simulink model "AD_Vehicle_part10"  (R2021a)
settings: Solver=VariableStepAuto  StartTime=0.0  StopTime=20  RelTol=1e-3
libraries: vrlib x2, mpcadaslib x1, pid_lib x1, simulink x1
settings Model: SimulationMode=accelerator  Creator=admin  LastModifiedBy=admin

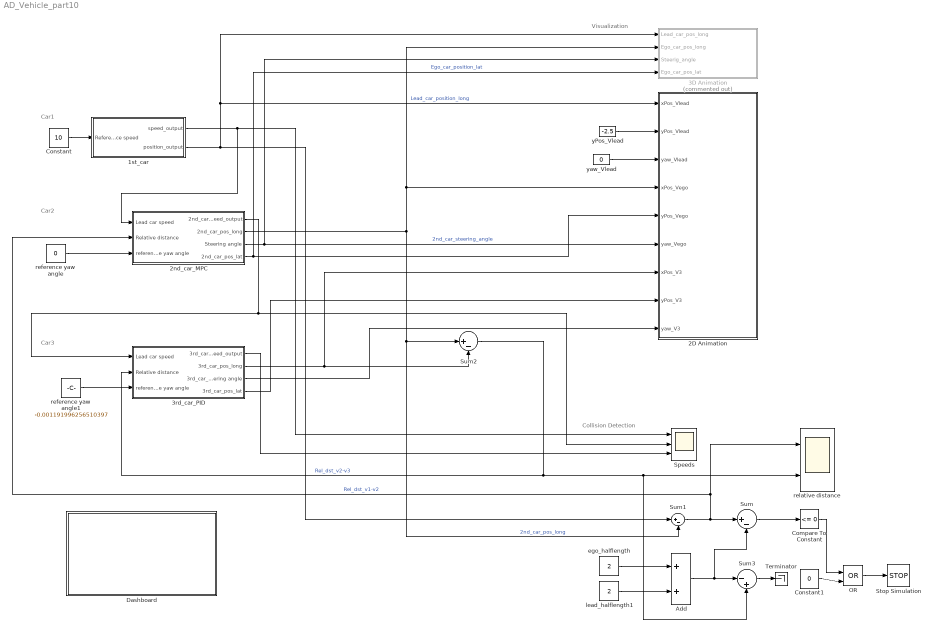
== system AD_Vehicle_part10 ==
  note: Car3
  note: Car2
  note: Car1
  note: Visualization
  note: Collision Detection
  1st_car : Subsystem  mask{Pos=40, Speed=20}
      mask prompts: Pos "Initial Position"; Speed "Initial Speed"
      mask TypeOptions Pos: initial_position/Value
      mask TypeOptions Speed: initial_speed/Value
  2D Animation : Subsystem  TreatAsAtomicUnit=on  SystemSampleTime=0.02
  2nd_car_MPC : Subsystem  mask{Pos_Z=20, Speed=25, Pos_X=-2.5}
      mask prompts: Pos_Z "Initial Position longi"; Speed "Initial Speed"; Pos_X "Initial position lat"
      mask TypeOptions Pos_Z: initial_position_long/Value
      mask TypeOptions Speed: initial_speed/Value
      mask TypeOptions Pos_X: initial_position_lat/Value
  3D Animation : Subsystem  Commented=on
  3rd_car_PID : Subsystem  mask{Pos_Z=0, Speed=20, Pos_X=-2.5}
      mask prompts: Pos_Z "Initial Position longi"; Speed "Initial Speed"; Pos_X "Initial position lat"
      mask TypeOptions Pos_Z: initial_position_long/Value
      mask TypeOptions Speed: initial_speed/Value
      mask TypeOptions Pos_X: initial_position_lat/Value
  Add : Sum
  Compare To Constant : simulink/Logic and Bit Operations/Compare To Constant  relop=<=  const=0  OutDataTypeStr=boolean
  Constant : Constant  Value=10
  Constant1 : Constant  Value=0
  Dashboard : Subsystem
  OR : Logic  Operator=OR  IconShape=distinctive  AllPortsSameDT=off  OutDataTypeStr=boolean
  Speeds : Scope  NumInputPorts=3
  Stop Simulation : Stop
  Sum : Sum  Inputs=|+-
  Sum1 : Sum  Inputs=|+-
  Sum2 : Sum  Inputs=|+-
  Sum3 : Sum  Inputs=|-+
  Terminator : Terminator
  ego_halflength : Constant  Value=2
  lead_halflength1 : Constant  Value=2
  reference yaw angle : Constant  Value=0
  reference yaw angle1 : Constant  Value=-0.001191996256510397
  relative distance : Scope  NumInputPorts=2
  yPos_Vlead : Constant  Value=-2.5
  yaw_Vlead : Constant  Value=0
  wires:
  3rd_car_PID/2(3rd_car_pos_long) -> 2D Animation/7(xPos_V3), Sum2/2
  Sum/1 -> Compare To Constant/1
  Constant/1 -> 1st_car/1(Reference speed)
  Sum2/1 -> Sum3/2, relative distance/2, 3rd_car_PID/2(Relative distance)  "Rel_dst_v2-v3"
  2nd_car_MPC/1(2nd_car_speed_output) -> 3rd_car_PID/1(Lead car speed), Speeds/2
  reference yaw angle1/1 -> 3rd_car_PID/3(reference yaw angle)
  2nd_car_MPC/4(2nd_car_pos_lat) -> 3D Animation/4(Ego_car_pos_lat), 2D Animation/5(yPos_Vego)  "Ego_car_position_lat"
  reference yaw angle/1 -> 2nd_car_MPC/3(reference yaw angle)
  Sum1/1 -> 2nd_car_MPC/2(Relative distance), relative distance/1, Sum/1  "Rel_dst_v1-v2"
  2nd_car_MPC/3(Steering angle) -> 3D Animation/3(Steerig_angle), 2D Animation/6(yaw_Vego)  "2nd_car_steering_angle"
  lead_halflength1/1 -> Add/2
  2nd_car_MPC/2(2nd_car_pos_long) -> Sum1/2, Sum2/1, 2D Animation/4(xPos_Vego), 3D Animation/2(Ego_car_pos_long)  "2nd_car_pos_long"
  yaw_Vlead/1 -> 2D Animation/3(yaw_Vlead)
  yPos_Vlead/1 -> 2D Animation/2(yPos_Vlead)
  1st_car/2(position_output) -> 3D Animation/1(Lead_car_pos_long), 2D Animation/1(xPos_Vlead), Sum1/1  "Lead_car_position_long"
  1st_car/1(speed_output) -> Speeds/1, 2nd_car_MPC/1(Lead car speed)
  Constant1/1 -> OR/2
  Sum3/1 -> Terminator/1
  Compare To Constant/1 -> OR/1
  Add/1 -> Sum3/1, Sum/2
  OR/1 -> Stop Simulation/1
  ego_halflength/1 -> Add/1
  3rd_car_PID/1(3rd_car_speed_output) -> Speeds/3
  3rd_car_PID/4(3rd_car_pos_lat) -> 2D Animation/8(yPos_V3)
  3rd_car_PID/3(3rd_car_Steering angle) -> 2D Animation/9(yaw_V3)

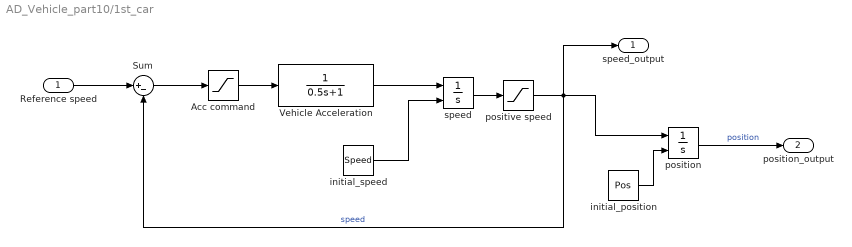
== system AD_Vehicle_part10/1st_car ==
  Reference speed : Inport
  Acc command : Saturate  UpperLimit=2  LowerLimit=-3
  Sum : Sum  Inputs=|+-
  Vehicle Acceleration : TransferFcn  Denominator=[0.5 1]
  initial_position : Constant  Value=Pos
  initial_speed : Constant  Value=Speed
  position : Integrator  InitialConditionSource=external
  positive speed : Saturate  UpperLimit=220  LowerLimit=0
  speed : Integrator  InitialConditionSource=external
  speed_output : Outport
  position_output : Outport  Port=2
  wires:
  Acc command/1 -> Vehicle Acceleration/1
  positive speed/1 -> speed_output/1, Sum/2, position/1  "speed"
  position/1 -> position_output/1  "position"
  speed/1 -> positive speed/1
  initial_position/1 -> position/2
  Sum/1 -> Acc command/1
  initial_speed/1 -> speed/2
  Reference speed/1 -> Sum/1
  Vehicle Acceleration/1 -> speed/1

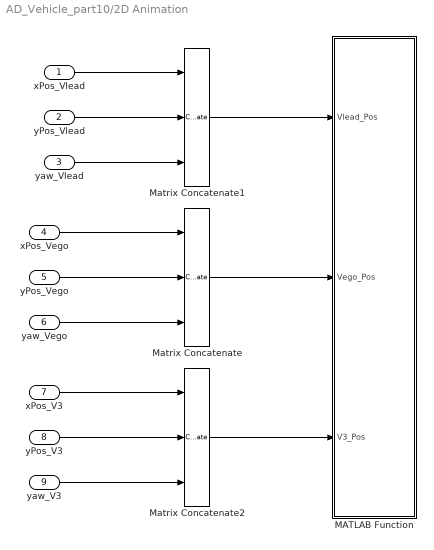
== system AD_Vehicle_part10/2D Animation ==
  xPos_Vlead : Inport
  yPos_Vlead : Inport  Port=2
  yaw_Vlead : Inport  Port=3
  xPos_Vego : Inport  Port=4
  yPos_Vego : Inport  Port=5
  yaw_Vego : Inport  Port=6
  xPos_V3 : Inport  Port=7
  yPos_V3 : Inport  Port=8
  yaw_V3 : Inport  Port=9
  MATLAB Function : MATLAB Function  TreatAsAtomicUnit=on
      mask init:
      | close all;
      | figure('units','normalized','outerposition',[0.5 0 0.5 1]); % 设置窗口(figure)位置大小
      | set (gca,'units','normalized','position',[0.1,0.3,0.9,0.5] ); % 设置画布(axis)大小位置
      | grid on;
      | axis equal;
      | hold on;
  Matrix Concatenate : Concatenate  NumInputs=3  ConcatenateDimension=2
  Matrix Concatenate1 : Concatenate  NumInputs=3  ConcatenateDimension=2
  Matrix Concatenate2 : Concatenate  NumInputs=3  ConcatenateDimension=2
  wires:
  Matrix Concatenate/1 -> MATLAB Function/2(Vego_Pos)
  yPos_Vego/1 -> Matrix Concatenate/2
  xPos_Vego/1 -> Matrix Concatenate/1
  yaw_Vego/1 -> Matrix Concatenate/3
  Matrix Concatenate1/1 -> MATLAB Function/1(Vlead_Pos)
  yPos_Vlead/1 -> Matrix Concatenate1/2
  xPos_Vlead/1 -> Matrix Concatenate1/1
  yaw_Vlead/1 -> Matrix Concatenate1/3
  xPos_V3/1 -> Matrix Concatenate2/1
  yPos_V3/1 -> Matrix Concatenate2/2
  yaw_V3/1 -> Matrix Concatenate2/3
  Matrix Concatenate2/1 -> MATLAB Function/3(V3_Pos)

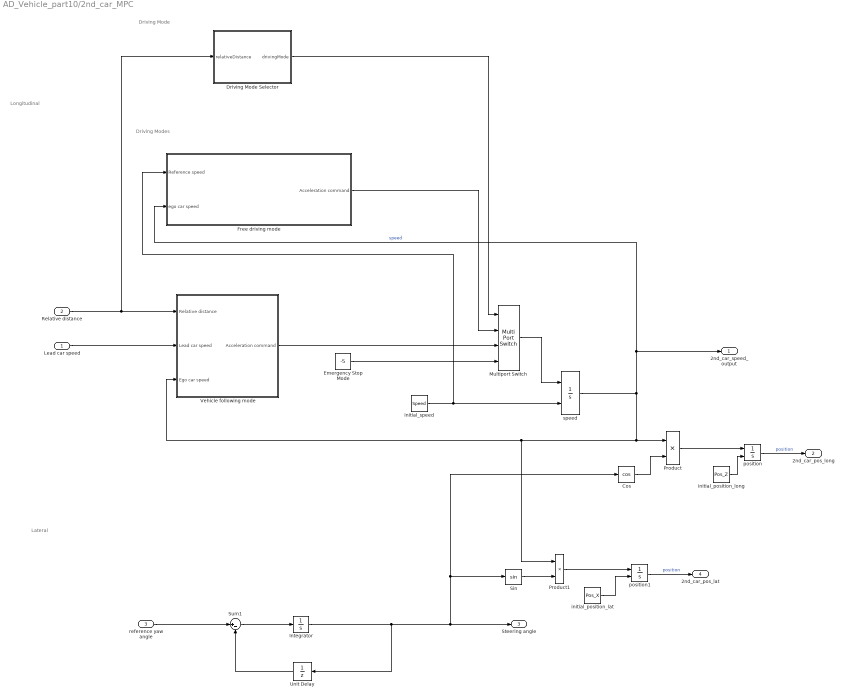
== system AD_Vehicle_part10/2nd_car_MPC ==
  note: Driving Mode
  note: Driving Modes
  note: Lateral
  note: Longitudinal
  Lead car speed : Inport
  Relative distance : Inport  Port=2
  reference yaw angle : Inport  Port=3
  Cos : Trigonometry  Operator=cos
  Driving Mode Selector : Stateflow chart  TreatAsAtomicUnit=on
  Emergency Stop Mode : Constant  Value=-5
  Free driving mode : Subsystem
  Integrator : Integrator
  Multiport Switch : MultiPortSwitch
  Product : Product
  Product1 : Product
  Sin : Trigonometry
  Sum1 : Sum  Inputs=|+-
  Unit Delay : UnitDelay  SampleTime=-1  HasFrameUpgradeWarning=on
  Vehicle following mode : Subsystem
  initial_position_lat : Constant  Value=Pos_X
  initial_position_long : Constant  Value=Pos_Z
  initial_speed : Constant  Value=Speed
  position : Integrator  InitialConditionSource=external
  position1 : Integrator  InitialConditionSource=external
  speed : Integrator  InitialConditionSource=external  LimitOutput=on  LowerSaturationLimit=0
  2nd_car_speed_output : Outport
  2nd_car_pos_long : Outport  Port=2
  Steering angle : Outport  Port=3
  2nd_car_pos_lat : Outport  Port=4
  wires:
  speed/1 -> Free driving mode/2("ego car speed "), 2nd_car_speed_output/1, Product1/1, Vehicle following mode/3(Ego car speed), Product/1  "speed"
  position/1 -> 2nd_car_pos_long/1  "position"
  initial_position_long/1 -> position/2
  initial_speed/1 -> speed/2, Free driving mode/1(Reference speed)
  Integrator/1 -> Unit Delay/1, Sin/1, Cos/1, Steering angle/1
  reference yaw angle/1 -> Sum1/1
  Sum1/1 -> Integrator/1
  Unit Delay/1 -> Sum1/2
  initial_position_lat/1 -> position1/2
  position1/1 -> 2nd_car_pos_lat/1  "position"
  Product/1 -> position/1
  Cos/1 -> Product/2
  Product1/1 -> position1/1
  Sin/1 -> Product1/2
  Relative distance/1 -> Vehicle following mode/1(Relative distance), Driving Mode Selector/1(relativeDistance)
  Lead car speed/1 -> Vehicle following mode/2(Lead car speed)
  Vehicle following mode/1(Acceleration command) -> Multiport Switch/3
  Multiport Switch/1 -> speed/1
  Free driving mode/1(Acceleration command) -> Multiport Switch/2
  Emergency Stop Mode/1 -> Multiport Switch/4
  Driving Mode Selector/1(drivingMode) -> Multiport Switch/1

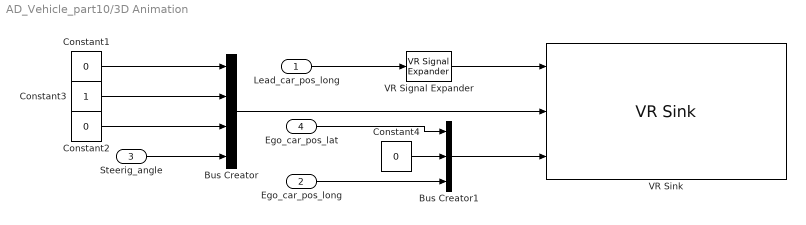
== system AD_Vehicle_part10/3D Animation ==
  Lead_car_pos_long : Inport
  Ego_car_pos_long : Inport  Port=2
  Steerig_angle : Inport  Port=3
  Ego_car_pos_lat : Inport  Port=4
  Bus Creator : BusCreator  Inputs=4
  Bus Creator1 : BusCreator  Inputs=3
  Constant1 : Constant  Value=0
  Constant2 : Constant  Value=0
  Constant3 : Constant
  Constant4 : Constant  Value=0
  VR Signal Expander : vrlib/VR Signal Expander  outwidth=3  outidx=[3]
  VR Sink : vrlib/VR Sink  InstantiateOnLoad=on  SampleTime=0.05  ViewEnable=on  RemoteChange=off  RemoteView=off  FieldsWritten=Car_Red.translation.3.1.1.double#Car_Blue.rotation.4.1.1.double#Car_Blue.translation.3.1.1.double  WorldFileName=PlatoonWorld.WRL  AutoView=off  VideoDimensions=[]  AllowVariableSize=off
  wires:
  Lead_car_pos_long/1 -> VR Signal Expander/1
  Constant4/1 -> Bus Creator1/2
  Bus Creator/1 -> VR Sink/2
  Constant1/1 -> Bus Creator/1
  Constant3/1 -> Bus Creator/2
  VR Signal Expander/1 -> VR Sink/1
  Ego_car_pos_long/1 -> Bus Creator1/3
  Bus Creator1/1 -> VR Sink/3
  Constant2/1 -> Bus Creator/3
  Ego_car_pos_lat/1 -> Bus Creator1/1
  Steerig_angle/1 -> Bus Creator/4

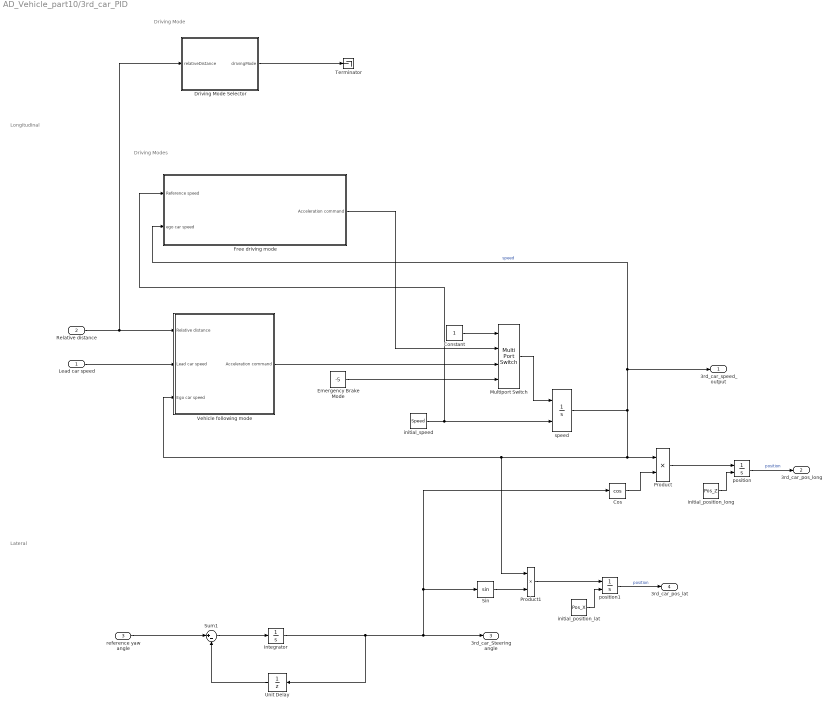
== system AD_Vehicle_part10/3rd_car_PID ==
  note: Driving Mode
  note: Driving Modes
  note: Lateral
  note: Longitudinal
  Lead car speed : Inport
  Relative distance : Inport  Port=2
  reference yaw angle : Inport  Port=3
  Constant : Constant
  Cos : Trigonometry  Operator=cos
  Driving Mode Selector : Stateflow chart  TreatAsAtomicUnit=on
  Emergency Brake Mode : Constant  Value=-5
  Free driving mode : Subsystem
  Integrator : Integrator
  Multiport Switch : MultiPortSwitch
  Product : Product
  Product1 : Product
  Sin : Trigonometry
  Sum1 : Sum  Inputs=|+-
  Terminator : Terminator
  Unit Delay : UnitDelay  SampleTime=-1  HasFrameUpgradeWarning=on
  Vehicle following mode : Subsystem
  initial_position_lat : Constant  Value=Pos_X
  initial_position_long : Constant  Value=Pos_Z
  initial_speed : Constant  Value=Speed
  position : Integrator  InitialConditionSource=external
  position1 : Integrator  InitialConditionSource=external
  speed : Integrator  InitialConditionSource=external  LimitOutput=on  LowerSaturationLimit=0
  3rd_car_speed_output : Outport
  3rd_car_pos_long : Outport  Port=2
  3rd_car_Steering angle : Outport  Port=3
  3rd_car_pos_lat : Outport  Port=4
  wires:
  speed/1 -> Free driving mode/2("ego car speed "), 3rd_car_speed_output/1, Product1/1, Vehicle following mode/3(Ego car speed), Product/1  "speed"
  position/1 -> 3rd_car_pos_long/1  "position"
  initial_position_long/1 -> position/2
  initial_speed/1 -> speed/2, Free driving mode/1(Reference speed)
  Integrator/1 -> Unit Delay/1, Sin/1, Cos/1, 3rd_car_Steering angle/1
  reference yaw angle/1 -> Sum1/1
  Sum1/1 -> Integrator/1
  Unit Delay/1 -> Sum1/2
  initial_position_lat/1 -> position1/2
  position1/1 -> 3rd_car_pos_lat/1  "position"
  Product/1 -> position/1
  Cos/1 -> Product/2
  Product1/1 -> position1/1
  Sin/1 -> Product1/2
  Relative distance/1 -> Vehicle following mode/1(Relative distance), Driving Mode Selector/1(relativeDistance)
  Lead car speed/1 -> Vehicle following mode/2(Lead car speed)
  Vehicle following mode/1(Acceleration command) -> Multiport Switch/3
  Multiport Switch/1 -> speed/1
  Free driving mode/1(Acceleration command) -> Multiport Switch/2
  Emergency Brake Mode/1 -> Multiport Switch/4
  Driving Mode Selector/1(drivingMode) -> Terminator/1
  Constant/1 -> Multiport Switch/1

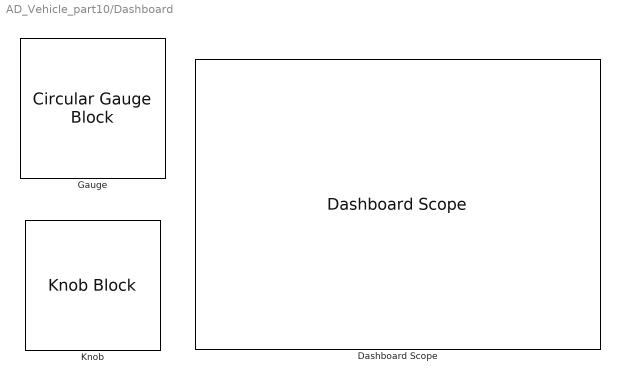
== system AD_Vehicle_part10/Dashboard ==
  Dashboard Scope : DashboardScope
  Gauge : CircularGaugeBlock  ScaleMax=180
  Knob : KnobBlock  ScaleMin=-0.2  ScaleMax=0.2

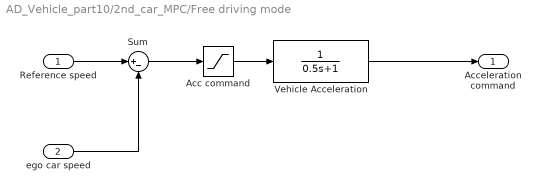
== system AD_Vehicle_part10/2nd_car_MPC/Free driving mode ==
  Reference speed : Inport
  "ego car speed " : Inport  Port=2
  Acc command : Saturate  UpperLimit=2  LowerLimit=-3
  Sum : Sum  Inputs=|+-
  Vehicle Acceleration : TransferFcn  Denominator=[0.5 1]
  Acceleration command : Outport
  wires:
  Vehicle Acceleration/1 -> Acceleration command/1
  Sum/1 -> Acc command/1
  Acc command/1 -> Vehicle Acceleration/1
  Reference speed/1 -> Sum/1
  "ego car speed "/1 -> Sum/2

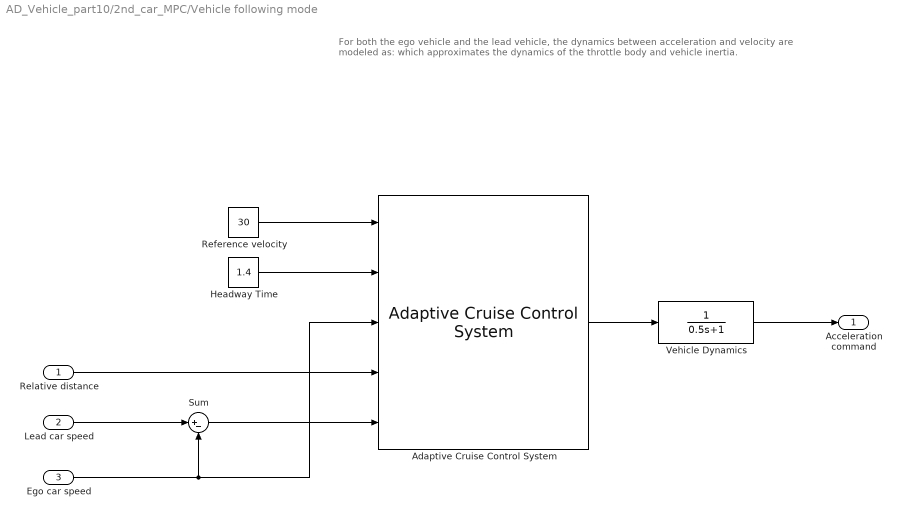
== system AD_Vehicle_part10/2nd_car_MPC/Vehicle following mode ==
  note: For both the ego vehicle and the lead vehicle, the dynamics between acceleration and velocity are modeled as:
      |
      | which approximates the dynamics of the throttle body and vehicle inertia.
  Relative distance : Inport
  Lead car speed : Inport  Port=2
  Ego car speed : Inport  Port=3
  Adaptive Cruise Control System : mpcadaslib/Adaptive Cruise Control System  EgoModel=tf(1,[0.5,1,0])  InitialEgoVelocity=30  DefaultSpacing=10  MaxVelocity=50  MinAcceleration=-3  amin_ext=off  MaxAcceleration=2  amax_ext=off  Ts=0.5  PredictionHorizon=200  ControllerBehavior=0.59  suboptimal=off  maxiter=10  datatypeopt=double  optmode=off  trackmode=off
  Headway Time : Constant  Value=1.4
  Reference velocity : Constant  Value=30
  Sum : Sum  Inputs=|+-
  Vehicle Dynamics : TransferFcn  Denominator=[0.5 1]
  Acceleration command : Outport
  wires:
  Vehicle Dynamics/1 -> Acceleration command/1
  Sum/1 -> Adaptive Cruise Control System/5
  Adaptive Cruise Control System/1 -> Vehicle Dynamics/1
  Headway Time/1 -> Adaptive Cruise Control System/2
  Lead car speed/1 -> Sum/1
  Reference velocity/1 -> Adaptive Cruise Control System/1
  Relative distance/1 -> Adaptive Cruise Control System/4
  Ego car speed/1 -> Adaptive Cruise Control System/3, Sum/2

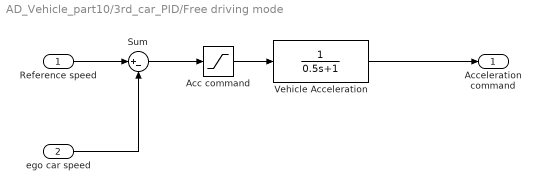
== system AD_Vehicle_part10/3rd_car_PID/Free driving mode ==
  Reference speed : Inport
  "ego car speed " : Inport  Port=2
  Acc command : Saturate  UpperLimit=2  LowerLimit=-3
  Sum : Sum  Inputs=|+-
  Vehicle Acceleration : TransferFcn  Denominator=[0.5 1]
  Acceleration command : Outport
  wires:
  Vehicle Acceleration/1 -> Acceleration command/1
  Sum/1 -> Acc command/1
  Acc command/1 -> Vehicle Acceleration/1
  Reference speed/1 -> Sum/1
  "ego car speed "/1 -> Sum/2

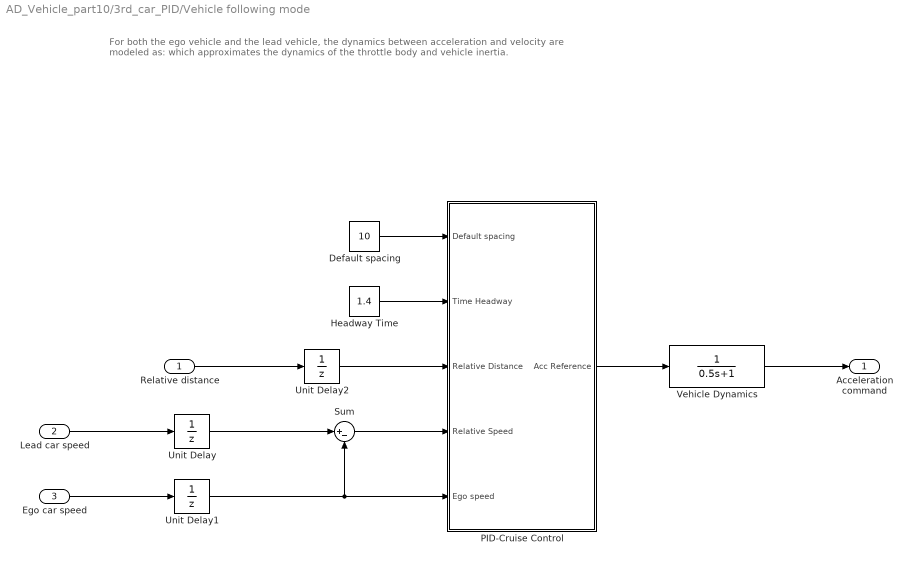
== system AD_Vehicle_part10/3rd_car_PID/Vehicle following mode ==
  note: For both the ego vehicle and the lead vehicle, the dynamics between acceleration and velocity are modeled as:
      |
      | which approximates the dynamics of the throttle body and vehicle inertia.
  Relative distance : Inport
  Lead car speed : Inport  Port=2
  Ego car speed : Inport  Port=3
  Default spacing : Constant  Value=10
  Headway Time : Constant  Value=1.4
  PID-Cruise Control : Subsystem
  Sum : Sum  Inputs=|+-
  Unit Delay : UnitDelay  SampleTime=-1  HasFrameUpgradeWarning=on
  Unit Delay1 : UnitDelay  SampleTime=-1  HasFrameUpgradeWarning=on
  Unit Delay2 : UnitDelay  SampleTime=-1  HasFrameUpgradeWarning=on
  Vehicle Dynamics : TransferFcn  Denominator=[0.5 1]
  Acceleration command : Outport
  wires:
  Vehicle Dynamics/1 -> Acceleration command/1
  Sum/1 -> PID-Cruise Control/4(Relative Speed)
  PID-Cruise Control/1(Acc Reference) -> Vehicle Dynamics/1
  Headway Time/1 -> PID-Cruise Control/2(Time Headway)
  Lead car speed/1 -> Unit Delay/1
  Default spacing/1 -> PID-Cruise Control/1(Default spacing)
  Ego car speed/1 -> Unit Delay1/1
  Unit Delay/1 -> Sum/1
  Unit Delay1/1 -> Sum/2, PID-Cruise Control/5(Ego speed)
  Unit Delay2/1 -> PID-Cruise Control/3(Relative Distance)
  Relative distance/1 -> Unit Delay2/1

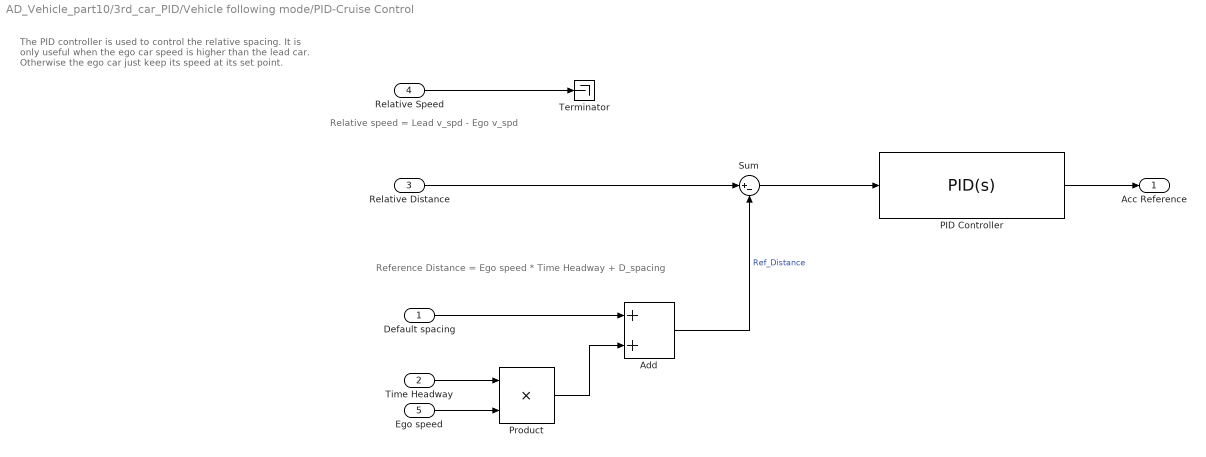
== system AD_Vehicle_part10/3rd_car_PID/Vehicle following mode/PID-Cruise Control ==
  note: The PID controller is used to control the relative spacing.
      | It is only useful when the ego car speed is higher than the lead car.
      | Otherwise the ego car just keep its speed at its set point.
  note: Relative speed = Lead v_spd - Ego v_spd
  note: Reference Distance = Ego speed * Time Headway + D_spacing
  Default spacing : Inport
  Time Headway : Inport  Port=2
  Relative Distance : Inport  Port=3
  Relative Speed : Inport  Port=4
  Ego speed : Inport  Port=5
  Add : Sum
  PID Controller : pid_lib/PID Controller  Controller=PID  Form=Parallel  TimeDomain=Continuous-time  UseExternalTs=off  SampleTime=-1  IntegratorMethod=Forward Euler  FilterMethod=Forward Euler  ControllerParametersSource=internal  P=2  I=0.04  D=2.1  UseFilter=on  N=230  TunerSelectOption=Transfer Function Based (PID Tuner App)  InitialConditionSource=internal  InitialConditionForIntegrator=0  InitialConditionForFilter=0  DifferentiatorICPrevScaledInput=0  ExternalReset=none  TrackingMode=off  Kt=1  LimitOutput=on  SatLimitsSource=internal  UpperSaturationLimit=2  LowerSaturationLimit=-3  LinearizeAsGain=on  AntiWindupMode=clamping  Kb=1  POutMin=[]  POutMax=[]  IOutMin=[]  IOutMax=[]  DOutMin=[]  DOutMax=[]  NOutMin=[]  NOutMax=[]  SumOutMin=[]  SumOutMax=[]  SaturationOutMin=[]  SaturationOutMax=[]  PParamMin=[]  PParamMax=[]  IParamMin=[]  IParamMax=[]  DParamMin=[]  DParamMax=[]  NParamMin=[]  NParamMax=[]  KbParamMin=[]  KbParamMax=[]  KtParamMin=[]  KtParamMax=[]  KbOutMin=[]  KbOutMax=[]  KtOutMin=[]  KtOutMax=[]  IntegratorOutMin=[]  IntegratorOutMax=[]  FilterOutMin=[]  FilterOutMax=[]  SumI1OutMin=[]  SumI1OutMax=[]  SumI2OutMin=[]  SumI2OutMax=[]  SumI3OutMin=[]  SumI3OutMax=[]  SumI4OutMin=[]  SumI4OutMax=[]  SumDOutMin=[]  SumDOutMax=[]  DifferentiatorOutMin=[]  DifferentiatorOutMax=[]  FilterDiffOutCoefMin=[]  FilterDiffOutCoefMax=[]  ReciprocalOutMin=[]  ReciprocalOutMax=[]  SumDenOutMin=[]  SumDenOutMax=[]  SumNumOutMin=[]  SumNumOutMax=[]  DivideOutMin=[]  DivideOutMax=[]  UdiffTsProdOutMin=[]  UdiffTsProdOutMax=[]  NTsProdOutMin=[]  NTsProdOutMax=[]  UintegralTsProdOutMin=[]  UintegralTsProdOutMax=[]  UngainTsProdOutMin=[]  UngainTsProdOutMax=[]  IntegratorContinuousStateAttributes=''  IntegratorStateMustResolveToSignalObject=off  IntegratorRTWStateStorageClass=Auto  FilterContinuousStateAttributes=''  FilterStateMustResolveToSignalObject=off  FilterRTWStateStorageClass=Auto  ParallelPVariant=InternalParameters  IdealPVariant=Disabled  IVariant=InternalParameters  DVariant=InternalParameters  IntegratorVariant=Continuous  SatVariant=Enabled  AWVariant=ContClampingParallel  PCopyVariant=Disabled  TRVariant=Disabled  FdbkBlocksVariant=Forward  IdealPFdbkVariant=Disabled  SatFdbkVariant=Disabled  DerivativeFilterVariant=ContFilter  NVariant=InternalParameters  NCopyVariant=Disabled  FilterICVariant=InternalICsFilter  IntegratorICVariant=InternalICs  ExternalResetVariant=Disabled  TRSumVariant=Passthrough  SumFdbkVariant=Disabled  SumVariant=Sum_PID  TsampFilterVariant=InternalTs  TsampNgainVariant=Passthrough  TsampIntegralVariant=Passthrough  ExternalSaturationOutDataTypeStr=Inherit: Same as second input
  Product : Product
  Sum : Sum  Inputs=|+-
  Terminator : Terminator
  Acc Reference : Outport
  wires:
  Time Headway/1 -> Product/1
  Ego speed/1 -> Product/2
  Default spacing/1 -> Add/1
  Product/1 -> Add/2
  Add/1 -> Sum/2  "Ref_Distance"
  Relative Distance/1 -> Sum/1
  Sum/1 -> PID Controller/1
  Relative Speed/1 -> Terminator/1
  PID Controller/1 -> Acc Reference/1

== stateflow chart AD_Vehicle_part10/3rd_car_PID/Driving Mode Selector ==
  state FreeDrivingMode
    entry:
    drivingMode = 1
  state FollowingMode
    entry:
    drivingMode = 2
  state EmergencyStop
    entry:
    drivingMode = 3
  (default) -> FreeDrivingMode
  FollowingMode -> FreeDrivingMode [order 1] : [relativeDistance > 50]
  FreeDrivingMode -> FollowingMode [order 1] : [relativeDistance <=0]
  FollowingMode -> EmergencyStop [order 2] : [relativeDistance <= 0]
  EmergencyStop -> FollowingMode : [relativeDistance > 15]
  FreeDrivingMode -> EmergencyStop [order 2] : [relativeDistance  <=0]
  data: relativeDistance input; drivingMode output

== matlab function AD_Vehicle_part10/2D Animation/MATLAB Function ==
  data: Vlead_Pos input; Vego_Pos input; V3_Pos input
function plotVehicle(Vlead_Pos,Vego_Pos, V3_Pos)
%% Clear previous Vehicles
cla;

%% Lead Vehicle - Position
x1 = Vlead_Pos(1);
y1 = Vlead_Pos(2);
yaw1 = Vlead_Pos(3);

LC_centerP = [x1;y1]; % 车辆质心位置

LC_halflength = 2;
LC_halfwidth = 1;

% Creating vehicle shape 定义矩形的四个顶点基于坐标原点的位置
LC_fl = [LC_halflength; LC_halfwidth]; % 车辆左前点
LC_fr = [LC_halflength; -LC_halfwidth]; % 车辆右前点
LC_rl = [-LC_halflength; LC_halfwidth]; % 车辆左后点
LC_rr = [-LC_halflength; -LC_halfwidth]; % 车辆右后点

% Final vehicle position 前车不考虑偏航
LC_flr = LC_centerP + LC_fl;
LC_frr = LC_centerP + LC_fr;
LC_rlr = LC_centerP + LC_rl;
LC_rrr = LC_centerP + LC_rr;

% Connecting points 将车辆四点连接起来形成代表车辆外形的矩形
Hitbox1 = [LC_flr LC_frr LC_rrr LC_rlr LC_flr]; % 2X5矩阵，第一行为各点横坐标，第二行为各点纵坐标
cornerLC_x = transpose(Hitbox1(1,:)); % 将横坐标保存为列向量
cornerLC_y = transpose(Hitbox1(2,:)); % 将纵坐标保存为列向量

%% Ego Vehicle - Position
x2 = Vego_Pos(1);
y2 = Vego_Pos(2);
yaw2 = Vego_Pos(3);

EC_centerP = [x2;y2]; % 车辆质心位置

EC_halflength = 2;
EC_halfwidth = 1;

% Creating vehicle shape 定义矩形的四个顶点基于坐标原点的位置
EC_fl = [EC_halflength; EC_halfwidth]; % 车辆左前点
EC_fr = [EC_halflength; -EC_halfwidth]; % 车辆右前点
EC_rl = [-EC_halflength; EC_halfwidth]; % 车辆左后点
EC_rr = [-EC_halflength; -EC_halfwidth]; % 车辆右后点

% Rotation Matrix 二维旋转矩阵
Mro2 = [cos(yaw2),-sin(yaw2);sin(yaw2),cos(yaw2)];

% Final vehicle position 考虑质心位置和偏航转角后的车辆四角坐标
EC_flr = EC_centerP + Mro2 * EC_fl;
EC_frr = EC_centerP + Mro2 * EC_fr;
EC_rlr = EC_centerP + Mro2 * EC_rl;
EC_rrr = EC_centerP + Mro2 * EC_rr;

% Connecting points 将车辆四点连接起来形成代表车辆外形的矩形
Hitbox2 = [EC_flr EC_frr EC_rrr EC_rlr EC_flr]; % 2X5矩阵，第一行为各点横坐标，第二行为各点纵坐标
cornerEC_x = transpose(Hitbox2(1,:)); % 将横坐标保存为列向量
cornerEC_y = transpose(Hitbox2(2,:)); % 将纵坐标保存为列向量

%% 3rd Vehicle - Position
x3 = V3_Pos(1);
y3 = V3_Pos(2);
yaw3 = V3_Pos(3);

V3_centerP = [x3;y3]; % 车辆质心位置

V3_halflength = 2;
V3_halfwidth = 1;

% Creating vehicle shape 定义矩形的四个顶点基于坐标原点的位置
V3_fl = [V3_halflength; V3_halfwidth]; % 车辆左前点
V3_fr = [V3_halflength; -V3_halfwidth]; % 车辆右前点
V3_rl = [-V3_halflength; V3_halfwidth]; % 车辆左后点
V3_rr = [-V3_halflength; -V3_halfwidth]; % 车辆右后点

% Rotation Matrix 二维旋转矩阵
Mro3 = [cos(yaw3),-sin(yaw3);sin(yaw3),cos(yaw3)];

% Final vehicle position 考虑质心位置和偏航转角后的车辆四角坐标
V3_flr = V3_centerP + Mro3 * V3_fl;
V3_frr = V3_centerP + Mro3 * V3_fr;
V3_rlr = V3_centerP + Mro3 * V3_rl;
V3_rrr = V3_centerP + Mro3 * V3_rr;

% Connecting points 将车辆四点连接起来形成代表车辆外形的矩形
Hitbox3 = [V3_flr V3_frr V3_rrr V3_rlr V3_flr]; % 2X5矩阵，第一行为各点横坐标，第二行为各点纵坐标
cornerV3_x = transpose(Hitbox3(1,:)); % 将横坐标保存为列向量
cornerV3_y = transpose(Hitbox3(2,:)); % 将纵坐标保存为列向量

%% Plot Vehicles and roads
plot(cornerLC_x,cornerLC_y,'r'); % 绘制代表Lead car的矩形
plot(x1,y1,'o'); % Lead car的质心

plot(cornerEC_x,cornerEC_y,'b'); % 绘制代表Ego car的矩形
plot(x2,y2,'*'); % 绘制Ego car的质心

plot(cornerV3_x,cornerV3_y,'g'); % 绘制代表3rd car的矩形
plot(x3,y3,'.'); % 绘制3rd car的质心

upperLine = plot([0 1000],[5 5],'color','black'); % 绘制上车道线
midLine = plot([0 1000],[0 0],'--','color','black'); % 绘制车道中线
lowerLine = plot([0 1000],[-5 -5],'color','black'); % 绘制下车道线

% Axis config
axis([x3-100 x3+100 y3-20 y3+20]); % 设置摄像头观察对象
%zoom yon;
zoom (1.5);

== stateflow chart AD_Vehicle_part10/2nd_car_MPC/Driving Mode Selector ==
  state FreeDrivingMode
    entry:
    drivingMode = 1
  state FollowingMode
    entry:
    drivingMode = 2
  state EmergencyStop
    entry:
    drivingMode = 3
  (default) -> FreeDrivingMode
  FollowingMode -> FreeDrivingMode [order 1] : [relativeDistance > 50]
  FreeDrivingMode -> FollowingMode [order 1] : [relativeDistance <=40]
  FollowingMode -> EmergencyStop [order 2] : [relativeDistance <= 10]
  EmergencyStop -> FollowingMode : [relativeDistance > 15]
  FreeDrivingMode -> EmergencyStop [order 2] : [relativeDistance  <=10]
  data: relativeDistance input; drivingMode output
